simulink model "step4_1_compare_lin_non_lin"  (R2022b)
settings: Solver=FixedStepAuto  StartTime=0.0  StopTime=RunTime  FixedStep=time_step  RelTol=1e-3
values from neighbouring files (symbols this model uses):
  A = [0 1 0 0 ... (first row only)    [linearize_script.m]    (also in step4_0_linearize_operating_point.m = double(A); step4_linearized_system.mat = [0 0.339319496362 0 -114.426616159 0 1 -102.612245897 0 221.; syms_test.m = double(A))
  B = [0 ... (first row only)    [linearize_script.m]    (also in step4_0_linearize_operating_point.m = double(B); step4_linearized_system.mat = [0 0 0 0 5076.90787281]; syms_test.m = double(B))
  C = [1 0 0 0 ... (first row only)    [linearize_script.m]    (also in matrixmaker_linearization.m = [b_1_0 - P_3 * theta_d_2 * sin(theta_2)  -P_3 * (theta_d_1 +; step4_0_linearize_operating_point.m = [1 0 0 0 0; step4_linearized_system.mat = [1  0  0  0  0; 0  0  1  0  0]; syms_test.m)
  D = zeros(2,1)    [linearize_script.m]    (also in step4_0_linearize_operating_point.m; step4_linearized_system.mat = [0 0]; syms_test.m)
  g1 = (m_1 * c_1_0 + m_2 * l_1) * g    [compare_ourmodel_with_others.m]    (also in step2_whitebox_beam.m; step4_0_linearize_operating_point.m; step5_observor_design.m; step6_1_controller_feedback.m)
  g2 = m_2 * c_2_0 * g    [compare_ourmodel_with_others.m]    (also in step2_whitebox_beam.m; step4_0_linearize_operating_point.m; step5_observor_design.m; step6_1_controller_feedback.m)
  P1 = m_1 * c_1_0 * c_1_0 + m_2 * l_1 * l_1 + I_1_0    [compare_ourmodel_with_others.m]    (also in script_for_test.m = P2(1:L/2+1); step2_whitebox_beam.m; step4_0_linearize_operating_point.m; step5_observor_design.m)
  P2 = m_2 * c_2_0 * c_2_0 + I_2_0    [compare_ourmodel_with_others.m]    (also in script_for_test.m = abs(Y/L); step2_whitebox_beam.m; step4_0_linearize_operating_point.m; step5_observor_design.m)
  P3 = m_2 * l_1 * c_2_0    [compare_ourmodel_with_others.m]    (also in step2_whitebox_beam.m; step4_0_linearize_operating_point.m; step5_observor_design.m; step6_1_controller_feedback.m)
  params = [9.81, 0.1, 0.1, 0.125, 0.05, -0.0300000121036330, 0.0813451968350115, 0.1000000000017210, 2.00882387117299e-05, 10.27570530021582, 2.78577414601457e-05, 65.9998023466922, 0.01300000000002200]    [compare_ourmodel_with_others.m]    (also in linearization.m = params_hat; matrixmaker_linearization.m = [-0.001, 0.077, 0.2, 0.00004, 20.684, 0.0004, 15, 0.03]; params.mat = [9.81 0.1 0.1 0.125 0.046955 -0.032 0.04609 0.0888 9.9e-05 6; sss.m = [9.81, 0.1, 0.1, 0.125, 0.04824, -0.041443, .0607558, 0.1154)
  theta_1_0 = pi    (= 3.14159265359)    [hwinit.m]    (also in hwinit_raw.m; step4_0_linearize_operating_point.m; step5_observor_design.m = x_op(1); step6_1_controller_feedback.m = x_op(1))
  theta_2_0 = 0    [hwinit.m]    (also in hwinit_raw.m; step4_0_linearize_operating_point.m; step5_observor_design.m = x_op(3); step6_1_controller_feedback.m = x_op(3))
  x_op = [theta_1_0; 0; theta_2_0; 0; 0]    [step4_0_linearize_operating_point.m]    (also in step4_linearized_system.mat = [3.14159265359 0 0 0 0])
settings Model: Creator=annel  LastModifiedBy=97083

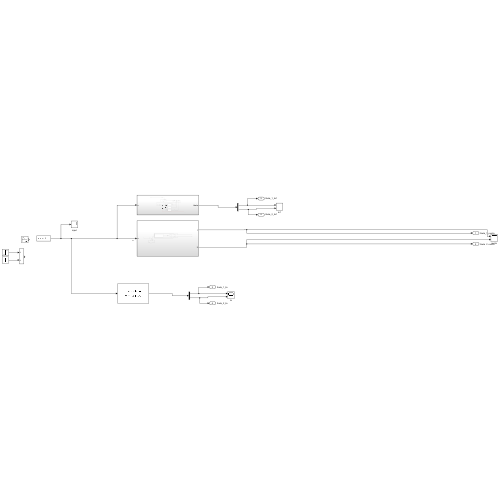
[thumbnail: Simulink's stored preview of the top-level diagram]
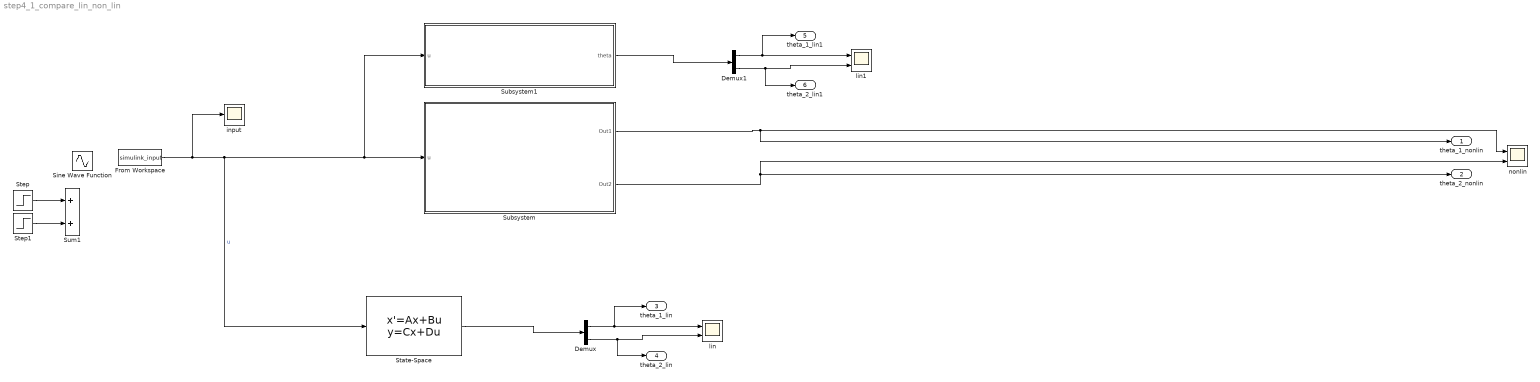
== system step4_1_compare_lin_non_lin ==
  Demux : Demux  Outputs=2
  Demux1 : Demux  Outputs=2
  From Workspace : FromWorkspace  SampleTime=-1
  Sine Wave Function : Sin  Amplitude=0.05  Frequency=2*pi*2  SampleTime=0.001
  State-Space : StateSpace  A=A  B=B  C=C  D=D  InitialCondition=x_op-x_op
  Step : Step  Time=0
  Step1 : Step  Time=0.05  After=-1
  Subsystem : Subsystem
  Subsystem1 : Subsystem
  Sum1 : Sum
  input : Scope
  lin : Scope  NumInputPorts=2
  lin1 : Scope  NumInputPorts=2
  nonlin : Scope  NumInputPorts=2
  theta_1_nonlin : Outport
  theta_2_nonlin : Outport  Port=2
  theta_1_lin : Outport  Port=3
  theta_2_lin : Outport  Port=4
  theta_1_lin1 : Outport  Port=5
  theta_2_lin1 : Outport  Port=6
  wires:
  Demux/1 -> theta_1_lin/1, lin/1
  Demux/2 -> lin/2, theta_2_lin/1
  State-Space/1 -> Demux/1
  Step1/1 -> Sum1/2
  Step/1 -> Sum1/1
  From Workspace/1 -> State-Space/1, Subsystem1/1(u), Subsystem/1(u), input/1  "u"
  Subsystem/1(Out1) -> theta_1_nonlin/1, nonlin/1
  Subsystem/2(Out2) -> nonlin/2, theta_2_nonlin/1
  Demux1/1 -> theta_1_lin1/1, lin1/1
  Demux1/2 -> lin1/2, theta_2_lin1/1
  Subsystem1/1(theta) -> Demux1/1

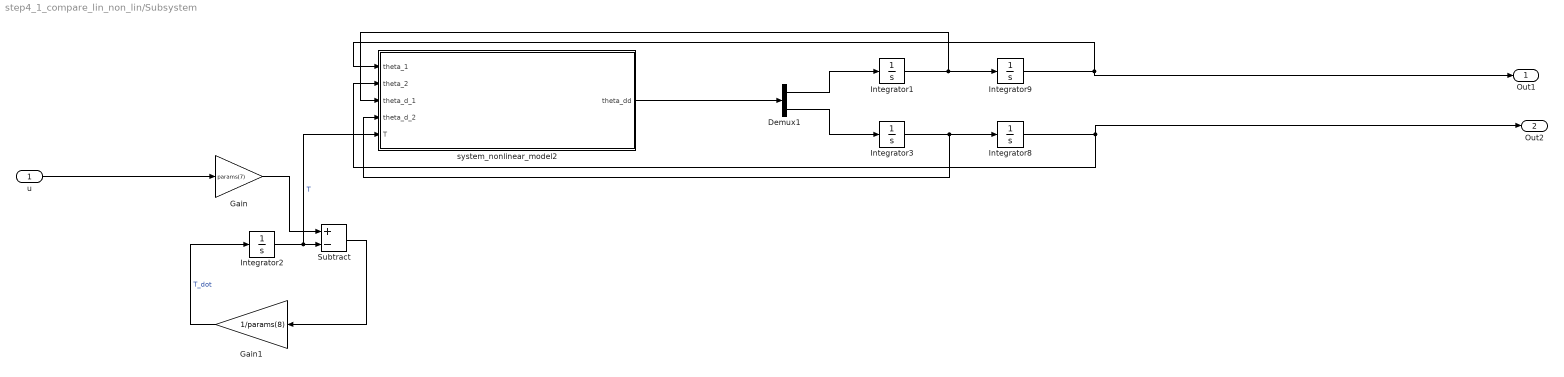
== system step4_1_compare_lin_non_lin/Subsystem ==
  u : Inport
  Demux1 : Demux  Outputs=2
  Gain : Gain  Gain=params(7)
  Gain1 : Gain  Gain=1/params(8)
  Integrator1 : Integrator
  Integrator2 : Integrator
  Integrator3 : Integrator
  Integrator8 : Integrator  InitialCondition=theta_2_0
  Integrator9 : Integrator  InitialCondition=theta_1_0
  Subtract : Sum  Inputs=+-
  system_nonlinear_model2 : MATLAB Function  TreatAsAtomicUnit=on
  Out1 : Outport
  Out2 : Outport  Port=2
  wires:
  Demux1/2 -> Integrator3/1
  Integrator1/1 -> system_nonlinear_model2/3(theta_d_1), Integrator9/1
  Integrator3/1 -> system_nonlinear_model2/4(theta_d_2), Integrator8/1
  system_nonlinear_model2/1(theta_dd) -> Demux1/1
  Integrator9/1 -> Out1/1, system_nonlinear_model2/1(theta_1)
  Integrator8/1 -> Out2/1, system_nonlinear_model2/2(theta_2)
  Subtract/1 -> Gain1/1
  Demux1/1 -> Integrator1/1
  Gain1/1 -> Integrator2/1  "T_dot"
  Gain/1 -> Subtract/1
  Integrator2/1 -> system_nonlinear_model2/5(T), Subtract/2  "T"
  u/1 -> Gain/1

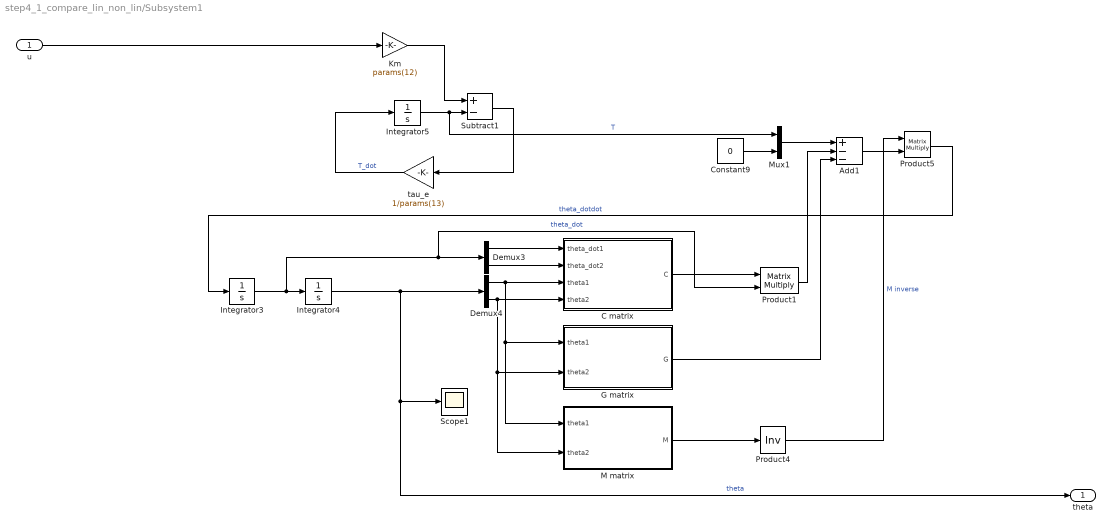
== system step4_1_compare_lin_non_lin/Subsystem1 ==
  u : Inport
  Add1 : Sum  Inputs=+--
  C matrix : MATLAB Function  TreatAsAtomicUnit=on
  Constant9 : Constant  Value=0
  Demux3 : Demux  Outputs=2
  Demux4 : Demux  Outputs=2
  G matrix : MATLAB Function  TreatAsAtomicUnit=on
  Integrator3 : Integrator
  Integrator4 : Integrator  InitialCondition=[theta_1_0, theta_2_0]
  Integrator5 : Integrator
  Km : Gain  Gain=params(12)
  M matrix : MATLAB Function  TreatAsAtomicUnit=on
  Mux1 : Mux  Inputs=2
  Product1 : Product  Inputs=**  Multiplication=Matrix(*)
  Product4 : Product  Inputs=/  Multiplication=Matrix(*)
  Product5 : Product  Inputs=**  Multiplication=Matrix(*)
  Scope1 : Scope
  Subtract1 : Sum  Inputs=+-
  tau_e : Gain  Gain=1/params(13)
  theta : Outport
  wires:
  Demux4/1 -> M matrix/1(theta1), G matrix/1(theta1), C matrix/3(theta1)
  tau_e/1 -> Integrator5/1  "T_dot"
  Constant9/1 -> Mux1/2
  Demux3/1 -> C matrix/1(theta_dot1)
  Add1/1 -> Product5/2
  Subtract1/1 -> tau_e/1
  G matrix/1(G) -> Add1/3
  Integrator3/1 -> Product1/2, Demux3/1, Integrator4/1  "theta_dot"
  C matrix/1(C) -> Product1/1
  Mux1/1 -> Add1/1
  Integrator5/1 -> Mux1/1, Subtract1/2  "T"
  u/1 -> Km/1
  Product5/1 -> Integrator3/1  "theta_dotdot"
  Demux3/2 -> C matrix/2(theta_dot2)
  Integrator4/1 -> Demux4/1, theta/1, Scope1/1  "theta"
  M matrix/1(M) -> Product4/1
  Demux4/2 -> M matrix/2(theta2), G matrix/2(theta2), C matrix/4(theta2)
  Product4/1 -> Product5/1  "M inverse"
  Product1/1 -> Add1/2
  Km/1 -> Subtract1/1

== matlab function step4_1_compare_lin_non_lin/Subsystem1/C matrix ==
  data: theta_dot1 input; theta_dot2 input; theta1 input; theta2 input; C output; params parameter; P3 parameter
function C = C(theta_dot1, theta_dot2, theta1, theta2, params, P3)
c00 = params(10) - P3 * theta_dot2 * sin(theta2);
c01 = -P3 * (theta_dot1 + theta_dot2) * sin(theta2);
c10 = P3 * theta_dot1 * sin(theta2);
c11 = params(11);

C = [c00 c01;
     c10 c11];

== matlab function step4_1_compare_lin_non_lin/Subsystem1/G matrix ==
  data: theta1 input; theta2 input; G output; g1 parameter; g2 parameter
function G = G(theta1, theta2, g1, g2)
G00 = -g1 * sin(theta1) - g2 * sin(theta1 + theta2);
G01 = -g2 * sin(theta1 + theta2);

G = [G00 G01];

== matlab function step4_1_compare_lin_non_lin/Subsystem1/M matrix ==
  data: theta1 input; theta2 input; M output; P1 parameter; P2 parameter; P3 parameter
function M = fcn(theta1, theta2, P1, P2, P3)
M00 = P1 + P2 + 2 * P3 * cos(theta2);
M01 = P2 + P3 * cos(theta2);
M10 = M01;
M11 = P2;

M = [M00 M01;
     M10 M11];

== matlab function step4_1_compare_lin_non_lin/Subsystem/system_nonlinear_model2 ==
  settings: updateMethod=DISCRETE  sampleTime=0.001
  data: theta_dd output size=2; theta_1 input size=1; theta_2 input size=1; theta_d_1 input size=1; theta_d_2 input size=1; T input size=1
function theta_dd    = get_theta_dt_dt(theta_1, theta_2, theta_d_1, theta_d_2, T)


% constant variables
g = 9.81;
l_1 = 0.1;
l_2 = 0.1;
m_1 = 0.125;
m_2 = 0.05;
% params = [-0.04, 0.06, 0.074, 0.00002, 4.8, 0.00077, 50, 0.03];
params = [0 -0.0300000121036330, 0.0813451968350115, 0.1000000000017210, 2.00882387117299e-05, 10.27570530021582, 2.78577414601457e-05, 65.9998023466922, 0.01300000000002200];


% varying variables

c_1_0 = params(2);
c_2_0 = params(3);
I_1_0 = params(4);
I_2_0 = params(5);
b_1_0 = params(6);
b_2_0 = params(7);
k_m_0 = params(8);
tau_e_0 = params(9);


theta_dd = [
                                                                                                                                          (2875084963116810*sin(theta_1 + theta_2)*(29307695852363*cos(theta_2) + 25287913028938))/(858941036174615393092683769*cos(theta_2)^2 - 183334706308915568681049596926) - (1822186171105643002107126611968*T)/(858941036174615393092683769*cos(theta_2)^2 - 183334706308915568681049596926) - theta_d_1*((1822186171105643002107126611968*((29307695852363*theta_d_2*sin(theta_2))/72057594037927936 - 5784707820127625/562949953421312))/(858941036174615393092683769*cos(theta_2)^2 - 183334706308915568681049596926) + (29307695852363*theta_d_1*sin(theta_2)*(29307695852363*cos(theta_2) + 25287913028938))/(858941036174615393092683769*cos(theta_2)^2 - 183334706308915568681049596926)) - (1822186171105643002107126611968*((1437542481558405*sin(theta_1 + theta_2))/36028797018963968 + (7068841419244153*sin(theta_1))/576460752303423488))/(858941036174615393092683769*cos(theta_2)^2 - 183334706308915568681049596926) - theta_d_2*((8222154034990009*(29307695852363*cos(theta_2) + 25287913028938))/(4096*(858941036174615393092683769*cos(theta_2)^2 - 183334706308915568681049596926)) + (1822186171105643002107126611968*sin(theta_2)*((29307695852363*theta_d_1)/72057594037927936 + (29307695852363*theta_d_2)/72057594037927936))/(858941036174615393092683769*cos(theta_2)^2 - 183334706308915568681049596926))
theta_d_1*((72057594037927936*((29307695852363*theta_d_2*sin(theta_2))/72057594037927936 - 5784707820127625/562949953421312)*(29307695852363*cos(theta_2) + 25287913028938))/(858941036174615393092683769*cos(theta_2)^2 - 183334706308915568681049596926) + (29307695852363*theta_d_1*sin(theta_2)*(58615391704726*cos(theta_2) + 7275182599835165))/(858941036174615393092683769*cos(theta_2)^2 - 183334706308915568681049596926)) + theta_d_2*((8222154034990009*(58615391704726*cos(theta_2) + 7275182599835165))/(4096*(858941036174615393092683769*cos(theta_2)^2 - 183334706308915568681049596926)) + (72057594037927936*sin(theta_2)*(29307695852363*cos(theta_2) + 25287913028938)*((29307695852363*theta_d_1)/72057594037927936 + (29307695852363*theta_d_2)/72057594037927936))/(858941036174615393092683769*cos(theta_2)^2 - 183334706308915568681049596926)) - (2875084963116810*sin(theta_1 + theta_2)*(58615391704726*cos(theta_2) + 7275182599835165))/(858941036174615393092683769*cos(theta_2)^2 - 183334706308915568681049596926) + (72057594037927936*T*(29307695852363*cos(theta_2) + 25287913028938))/(858941036174615393092683769*cos(theta_2)^2 - 183334706308915568681049596926) + (72057594037927936*(29307695852363*cos(theta_2) + 25287913028938)*((1437542481558405*sin(theta_1 + theta_2))/36028797018963968 + (7068841419244153*sin(theta_1))/576460752303423488))/(858941036174615393092683769*cos(theta_2)^2 - 183334706308915568681049596926);
];
